simulink model "vehicle_longitudinal_model"  (Simulink 8.9)
settings: Solver=ode23s  StartTime=0.0  StopTime=10.0  RelTol=1e-3  EnableMultiTasking=on
values from neighbouring files (symbols this model uses):
  c_aero = 0.53    [Setup_Lincoln_model.m]
  delay_brake = 0.2    [Setup_Lincoln_model.m]
  F_roll = 172    [Setup_Lincoln_model.m]
  h = h_v    (= 0.33)    [Setup_Lincoln_model.m]
  I_e = 0.2630    (= 0.263)    [Setup_Lincoln_model.m]
  I_wheel = 1.93    [Setup_Lincoln_model.m]
  KB = 0.9    [Setup_Lincoln_model.m]
  mass = 2000    [Setup_Lincoln_model.m]
  max_throttle = max(throttle_table)    [Setup_Lincoln_model.m]
  max_throttle_rate = 450    [Setup_Lincoln_model.m]
  min_throttle = min(throttle_table)    [Setup_Lincoln_model.m]
  mu_B = 22+(Fz-1940)/645    (= 26.5968992248)    [Setup_Lincoln_model.m]
  mu_C = 1.35-(Fz-1940)/16125    (= 1.16612403101)    [Setup_Lincoln_model.m]
  mu_D = 2000+(Fz-1940)/0.956    (= 5101.46443515)    [Setup_Lincoln_model.m]
  mu_E = -3.6    [Setup_Lincoln_model.m]
  P_po = 10.67    [Setup_Lincoln_model.m]
  Rdrive = 0.3058    [Setup_Lincoln_model.m]
  tau_brake = 0.1    [Setup_Lincoln_model.m]
  tau_throttle = 0.01    [Setup_Lincoln_model.m]
  throttle_o = 2    [Setup_Lincoln_model.m]
  w_wheel_o = x_dot_o/he    (= 63.6363636364)    [Setup_Lincoln_model.m]
  we_max = max(we_table)    [Setup_Lincoln_model.m]
  we_min = min(we_table)    [Setup_Lincoln_model.m]
  we_o = x_dot_o/(he*Rdrive*gear_ratios(3))    [Setup_Lincoln_model.m]
  x_dot_o = 21    [Setup_Lincoln_model.m]
undefined symbols (not defined in the file or in its folder): tnet_table
libraries: simulink x2
settings Model: Creator=user  LastModifiedBy=edward
settings OptimizationCC: ExpressionDepthLimit=2147483647  InitFltsAndDblsToZero=on
settings DebuggingCC: SolverPrmCheckMsg=warning  FcnCallInpInsideContextMsg=error
settings GRTTargetCC: GeneratePreprocessorConditionals=Use local settings

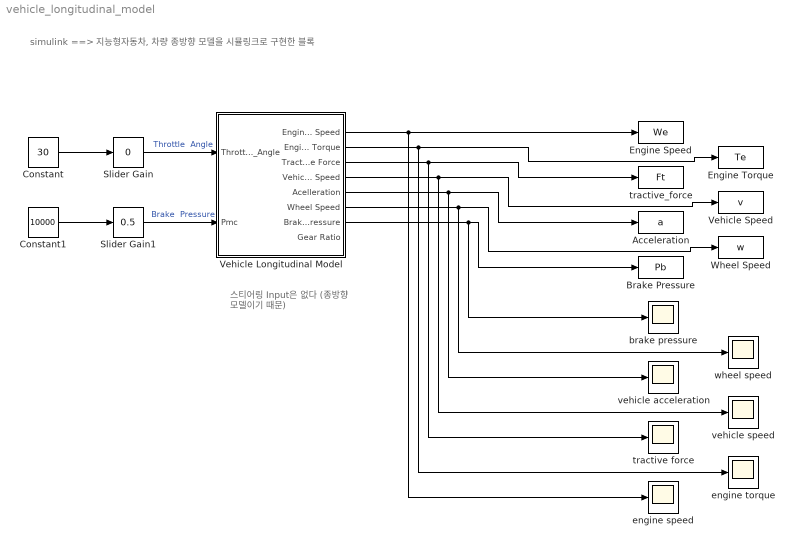
== system vehicle_longitudinal_model ==
  note: simulink ==> 지능형자동차, 차량 종방향 모델을 시뮬링크로 구현한 블록
  note: 스티어링 Input은 없다
      | (종방향 모델이기 때문)
  Acceleration : ToWorkspace  VariableName=a  SampleTime=-1
  Brake Pressure : ToWorkspace  VariableName=Pb  SampleTime=-1
  Constant : Constant  Value=30
  Constant1 : Constant  Value=10000
  Engine Speed : ToWorkspace  VariableName=We  SampleTime=-1
  Engine Torque : ToWorkspace  VariableName=Te  SampleTime=-1
  Slider Gain : simulink/Math Operations/Slider Gain  gain=0  low=0  high=1
  Slider Gain1 : simulink/Math Operations/Slider Gain  gain=0.5  low=0  high=1
  Vehicle Longitudinal Model : Subsystem
  Vehicle Speed : ToWorkspace  VariableName=v  SampleTime=-1
  Wheel Speed : ToWorkspace  VariableName=w  SampleTime=-1
  brake pressure : Scope
  engine speed : Scope
  engine torque : Scope
  tractive force : Scope
  tractive_force : ToWorkspace  VariableName=Ft  SampleTime=-1
  vehicle acceleration : Scope
  vehicle speed : Scope
  wheel speed : Scope
  wires:
  Constant/1 -> Slider Gain/1
  Slider Gain/1 -> Vehicle Longitudinal Model/1(Throttle_Angle)  "Throttle  Angle"
  Constant1/1 -> Slider Gain1/1
  Slider Gain1/1 -> Vehicle Longitudinal Model/2(Pmc)  "Brake  Pressure"
  Vehicle Longitudinal Model/1(Engine Speed) -> Engine Speed/1, engine speed/1
  Vehicle Longitudinal Model/3(Tractive Force) -> tractive force/1, tractive_force/1
  Vehicle Longitudinal Model/4(Vehicle Speed) -> Vehicle Speed/1, vehicle speed/1
  Vehicle Longitudinal Model/5(Acelleration) -> vehicle acceleration/1, Acceleration/1
  Vehicle Longitudinal Model/6(Wheel Speed) -> Wheel Speed/1, wheel speed/1
  Vehicle Longitudinal Model/7(Brake Pressure) -> brake pressure/1, Brake Pressure/1
  Vehicle Longitudinal Model/2(Engine Torque) -> Engine Torque/1, engine torque/1

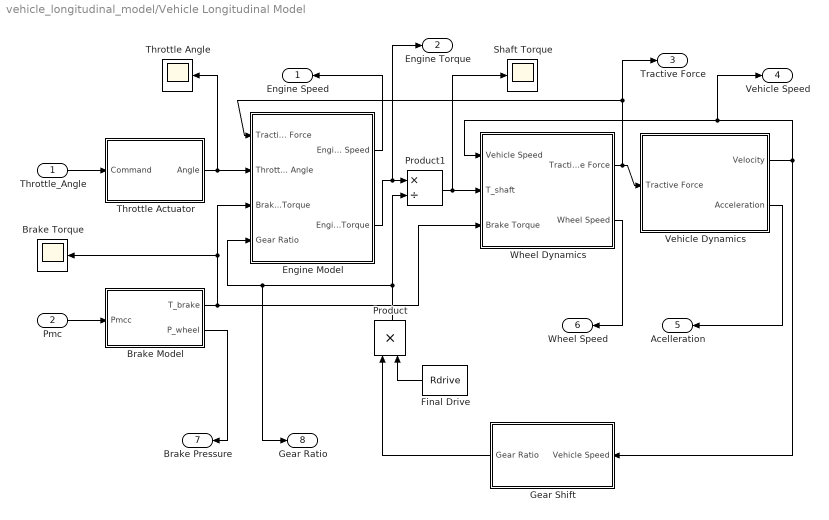
== system vehicle_longitudinal_model/Vehicle Longitudinal Model ==
  Throttle_Angle : Inport
  Pmc : Inport  Port=2
  Brake Model : Subsystem
  Brake Torque : Scope
  Engine Model : Subsystem
  Final Drive : Constant  Value=Rdrive
  Gear Shift : Subsystem
  Product : Product  Inputs=**  SaturateOnIntegerOverflow=on  RndMeth=Zero  InputSameDT=on  OutDataTypeStr=Inherit: Same as first input
  Product1 : Product  Inputs=*/  SaturateOnIntegerOverflow=on  RndMeth=Zero  InputSameDT=on  OutDataTypeStr=Inherit: Same as first input
  Shaft Torque : Scope
  Throttle Actuator : Subsystem
  Throttle Angle : Scope
  Vehicle Dynamics : Subsystem
  Wheel Dynamics : Subsystem
  Engine Speed : Outport
  Engine Torque : Outport  Port=2
  Tractive Force : Outport  Port=3
  Vehicle Speed : Outport  Port=4
  Acelleration : Outport  Port=5
  Wheel Speed : Outport  Port=6
  Brake Pressure : Outport  Port=7
  Gear Ratio : Outport  Port=8
  wires:
  Product1/1 -> Shaft Torque/1, Wheel Dynamics/2(T_shaft)
  Engine Model/2(Engine Torque) -> Product1/1, Engine Torque/1
  Engine Model/1(Engine Speed) -> Engine Speed/1
  Brake Model/1(T_brake) -> Engine Model/3(Brake Torque), Brake Torque/1, Wheel Dynamics/3(Brake Torque)
  Product/1 -> Product1/2, Engine Model/4(Gear Ratio), Gear Ratio/1
  Final Drive/1 -> Product/2
  Gear Shift/1(Gear Ratio) -> Product/1
  Wheel Dynamics/1(Tractive Force) -> Vehicle Dynamics/1(Tractive Force), Engine Model/1(Tractive Force), Tractive Force/1
  Throttle Actuator/1(Angle) -> Engine Model/2(Throttle Angle), Throttle Angle/1
  Throttle_Angle/1 -> Throttle Actuator/1(Command)
  Pmc/1 -> Brake Model/1(Pmcc)
  Brake Model/2(P_wheel) -> Brake Pressure/1
  Vehicle Dynamics/1(Velocity) -> Vehicle Speed/1, Wheel Dynamics/1(Vehicle Speed), Gear Shift/1(Vehicle Speed)
  Vehicle Dynamics/2(Acceleration) -> Acelleration/1
  Wheel Dynamics/2(Wheel Speed) -> Wheel Speed/1

== system vehicle_longitudinal_model/Vehicle Longitudinal Model/Brake Model ==
  note: Wheel Pressure가 브레이크 패드에 있는
      | Spring(k)보다 크게 걸렸을 때에만 브레이크가 작동하므로
      | Dead Zone이 발생한다
  note: Wheel pressure
  note: brake는 1차 전달함수의 response를 보인다
  note: Valve를 여닫는 시간에 따라
      | 필연적으로 발생하는 Time Delay
  Pmcc : Inport
  Brake Coefficient : Gain  Gain=KB  SaturateOnIntegerOverflow=on  OutDataTypeStr=Inherit: Same as input  ParamDataTypeStr=Inherit: Same as input
  Brake Dynamics : TransferFcn  Denominator=[tau_brake 1]
  Dead Zone : DeadZone  LowerValue=-P_po  UpperValue=P_po  SaturateOnIntegerOverflow=on
  Pure Time Delay : TransportDelay  DelayTime=delay_brake
  T_brake : Outport
  P_wheel : Outport  Port=2
  wires:
  Brake Coefficient/1 -> T_brake/1
  Dead Zone/1 -> Brake Coefficient/1
  Brake Dynamics/1 -> P_wheel/1, Dead Zone/1  "P_wheel"
  Pmcc/1 -> Pure Time Delay/1
  Pure Time Delay/1 -> Brake Dynamics/1

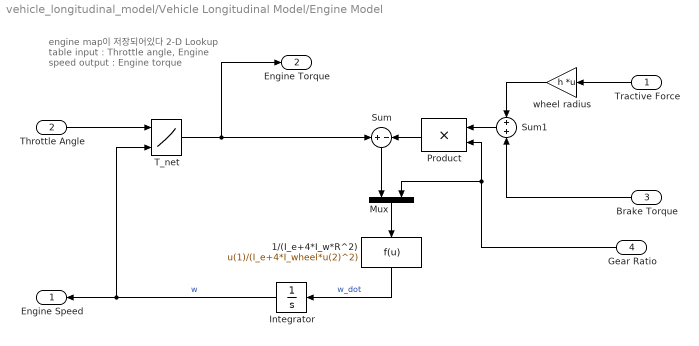
== system vehicle_longitudinal_model/Vehicle Longitudinal Model/Engine Model ==
  note: engine map이 저장되어있다
      | 2-D Lookup table
      |
      | input : Throttle angle, Engine speed
      | output : Engine torque
  Tractive Force : Inport
  Throttle Angle : Inport  Port=2
  Brake Torque : Inport  Port=3
  Gear Ratio : Inport  Port=4
  1/(I_e+4*I_w*R^2) : Fcn  Expr=u(1)/(I_e+4*I_wheel*u(2)^2)
  Integrator : Integrator  InitialCondition=we_o  LimitOutput=on  UpperSaturationLimit=[we_max]  LowerSaturationLimit=[we_min]
  Mux : Mux  Inputs=2
  Product : Product  SaturateOnIntegerOverflow=on  RndMeth=Zero  InputSameDT=on  OutDataTypeStr=Inherit: Same as first input
  Sum : Sum  Inputs=+|-  SaturateOnIntegerOverflow=on  InputSameDT=on  OutDataTypeStr=Inherit: Same as first input
  Sum1 : Sum  SaturateOnIntegerOverflow=on  InputSameDT=on  OutDataTypeStr=Inherit: Same as first input
  T_net : Lookup2D  RowIndex=alpha_table  ColumnIndex=we_table  Table=tnet_table  SaturateOnIntegerOverflow=on  InputSameDT=on
  wheel radius : Gain  Gain=h  Multiplication=Matrix(K*u)  SaturateOnIntegerOverflow=on  OutDataTypeStr=Inherit: Same as input  ParamDataTypeStr=Inherit: Same as input
  Engine Speed : Outport
  Engine Torque : Outport  Port=2
  wires:
  Throttle Angle/1 -> T_net/1
  Integrator/1 -> Engine Speed/1, T_net/2  "w"
  1/(I_e+4*I_w*R^2)/1 -> Integrator/1  "w_dot"
  Tractive Force/1 -> wheel radius/1
  wheel radius/1 -> Sum1/1
  Brake Torque/1 -> Sum1/2
  Product/1 -> Sum/2
  Sum1/1 -> Product/1
  Gear Ratio/1 -> Product/2, Mux/2
  Sum/1 -> Mux/1
  Mux/1 -> 1/(I_e+4*I_w*R^2)/1
  T_net/1 -> Engine Torque/1, Sum/1

== system vehicle_longitudinal_model/Vehicle Longitudinal Model/Gear Shift ==
  note: [1 1 1]인 [n,1] 행렬과
      | 반환행렬을 곱해서
      | 스칼라값(기어값)을 만든다
  note: 현재 차량 속도 vs 기어변속 속도를 비교한다
      | [0; 1; 1] 같은 [1,n]행렬이 반환된다
  Vehicle Speed : Inport
  Convert m/s to mph : Gain  Gain=3.6/1.6  SaturateOnIntegerOverflow=on  OutDataTypeStr=Inherit: Same as input  ParamDataTypeStr=Inherit: Same as input
  Direct Look-Up of Gear ratio : LookupNDDirect  NumberOfTableDimensions=1  Table=[0.3423,0.6378,1.0,1.4184]
  Get gear-1 : Gain  Gain=ones(1,3)  Multiplication=Matrix(K*u)  SaturateOnIntegerOverflow=on  OutDataTypeStr=Inherit: Same as input  ParamDataTypeStr=Inherit: Same as input
  Relational Operator : RelationalOperator  Operator=>  RndMeth=Nearest  InputSameDT=on
  Shift Speeds : Constant  Value=[15 32 67]
  Gear Ratio : Outport
  wires:
  Shift Speeds/1 -> Relational Operator/2
  Relational Operator/1 -> Get gear-1/1
  Convert m/s to mph/1 -> Relational Operator/1
  Get gear-1/1 -> Direct Look-Up of Gear ratio/1
  Vehicle Speed/1 -> Convert m/s to mph/1
  Direct Look-Up of Gear ratio/1 -> Gear Ratio/1

== system vehicle_longitudinal_model/Vehicle Longitudinal Model/Throttle Actuator ==
  Command : Inport
  Integrator : Integrator  InitialCondition=throttle_o  LimitOutput=on  UpperSaturationLimit=max_throttle  LowerSaturationLimit=min_throttle
  Saturation : Saturate  UpperLimit=max_throttle_rate  LowerLimit=-max_throttle_rate
  Sum : Sum  Inputs=-+|  SaturateOnIntegerOverflow=on  InputSameDT=on  OutDataTypeStr=Inherit: Same as first input
  Throttle Time Constant : Gain  Gain=1/tau_throttle  SaturateOnIntegerOverflow=on  OutDataTypeStr=Inherit: Same as input  ParamDataTypeStr=Inherit: Same as input
  Angle : Outport
  wires:
  Command/1 -> Sum/2
  Integrator/1 -> Angle/1, Sum/1
  Sum/1 -> Throttle Time Constant/1
  Throttle Time Constant/1 -> Saturation/1
  Saturation/1 -> Integrator/1

== system vehicle_longitudinal_model/Vehicle Longitudinal Model/Vehicle Dynamics ==
  note: 타이어저항 F_road
  note: v
  note: v_dot
  note: 공기저항 F_air
  note: 구름저항 F_roll
  Tractive Force : Inport
  Aerodynamic Drag : Fcn  Expr=c_aero*u^2
  Divide by Mass : Gain  Gain=1/mass  Multiplication=Matrix(K*u)  SaturateOnIntegerOverflow=on  OutDataTypeStr=Inherit: Same as input  ParamDataTypeStr=Inherit: Same as input
  Integrator : Integrator  InitialCondition=x_dot_o  LimitOutput=on  LowerSaturationLimit=0
  Rolling Resistance : Constant  Value=F_roll
  Sum1 : Sum  Inputs=--+  SaturateOnIntegerOverflow=on  InputSameDT=on  OutDataTypeStr=Inherit: Same as first input
  Velocity : Outport
  Acceleration : Outport  Port=2
  wires:
  Tractive Force/1 -> Sum1/3
  Divide by Mass/1 -> Acceleration/1, Integrator/1
  Integrator/1 -> Velocity/1, Aerodynamic Drag/1
  Sum1/1 -> Divide by Mass/1
  Rolling Resistance/1 -> Sum1/2
  Aerodynamic Drag/1 -> Sum1/1

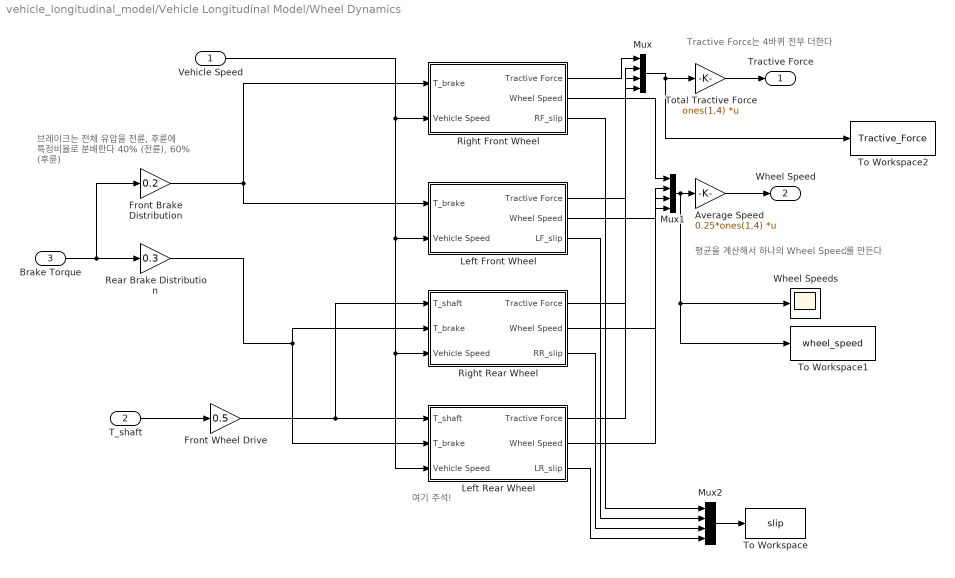
== system vehicle_longitudinal_model/Vehicle Longitudinal Model/Wheel Dynamics ==
  note: 여기 주석!
  note: Tractive Force는 4바퀴 전부 더한다
  note: 평균을 계산해서 하나의 Wheel Speed를 만든다
  note: 브레이크는 전체 유압을
      | 전륜, 후륜에 특정비율로 분배한다
      | 40% (전륜), 60% (후륜)
  Vehicle Speed : Inport
  T_shaft : Inport  Port=2
  Brake Torque : Inport  Port=3
  Average Speed : Gain  Gain=0.25*ones(1,4)  Multiplication=Matrix(K*u)  SaturateOnIntegerOverflow=on  OutDataTypeStr=Inherit: Same as input  ParamDataTypeStr=Inherit: Same as input
  Front Brake Distribution : Gain  Gain=0.2  SaturateOnIntegerOverflow=on  OutDataTypeStr=Inherit: Same as input  ParamDataTypeStr=Inherit: Same as input
  Front Wheel Drive : Gain  Gain=0.5  SaturateOnIntegerOverflow=on  OutDataTypeStr=Inherit: Same as input  ParamDataTypeStr=Inherit: Same as input
  Left Front Wheel : Subsystem
  Left Rear Wheel : Subsystem
  Mux : Mux
  Mux1 : Mux
  Mux2 : Mux
  Rear Brake Distribution : Gain  Gain=0.3  SaturateOnIntegerOverflow=on  OutDataTypeStr=Inherit: Same as input  ParamDataTypeStr=Inherit: Same as input
  Right Front Wheel : Subsystem
  Right Rear Wheel : Subsystem
  To Workspace : ToWorkspace  VariableName=slip  SampleTime=-1
  To Workspace1 : ToWorkspace  VariableName=wheel_speed  SampleTime=-1
  To Workspace2 : ToWorkspace  VariableName=Tractive_Force  SampleTime=-1
  Total Tractive Force : Gain  Gain=ones(1,4)  Multiplication=Matrix(K*u)  SaturateOnIntegerOverflow=on  OutDataTypeStr=Inherit: Same as input  ParamDataTypeStr=Inherit: Same as input
  Wheel Speeds : Scope
  Tractive Force : Outport
  Wheel Speed : Outport  Port=2
  wires:
  Total Tractive Force/1 -> Tractive Force/1
  Average Speed/1 -> Wheel Speed/1
  Mux/1 -> Total Tractive Force/1, To Workspace2/1
  Vehicle Speed/1 -> Right Front Wheel/2(Vehicle Speed), Left Rear Wheel/3(Vehicle Speed), Right Rear Wheel/3(Vehicle Speed), Left Front Wheel/2(Vehicle Speed)
  Right Front Wheel/1(Tractive Force) -> Mux/1
  Left Front Wheel/1(Tractive Force) -> Mux/2
  Right Rear Wheel/1(Tractive Force) -> Mux/3
  Left Rear Wheel/1(Tractive Force) -> Mux/4
  Mux1/1 -> Average Speed/1, Wheel Speeds/1, To Workspace1/1
  Right Front Wheel/2(Wheel Speed) -> Mux1/1
  Left Front Wheel/2(Wheel Speed) -> Mux1/2
  Right Rear Wheel/2(Wheel Speed) -> Mux1/3
  Left Rear Wheel/2(Wheel Speed) -> Mux1/4
  Right Front Wheel/3(RF_slip) -> Mux2/1
  Left Rear Wheel/3(LR_slip) -> Mux2/4
  Mux2/1 -> To Workspace/1
  T_shaft/1 -> Front Wheel Drive/1
  Front Wheel Drive/1 -> Right Rear Wheel/1(T_shaft), Left Rear Wheel/1(T_shaft)
  Brake Torque/1 -> Rear Brake Distribution/1, Front Brake Distribution/1
  Left Front Wheel/3(LF_slip) -> Mux2/2
  Right Rear Wheel/3(RR_slip) -> Mux2/3
  Front Brake Distribution/1 -> Right Front Wheel/1(T_brake), Left Front Wheel/1(T_brake)
  Rear Brake Distribution/1 -> Left Rear Wheel/2(T_brake), Right Rear Wheel/2(T_brake)

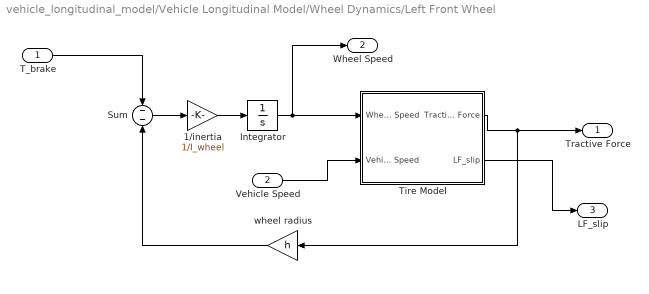
== system vehicle_longitudinal_model/Vehicle Longitudinal Model/Wheel Dynamics/Left Front Wheel ==
  T_brake : Inport
  Vehicle Speed : Inport  Port=2
  1/inertia : Gain  Gain=1/I_wheel  SaturateOnIntegerOverflow=on  OutDataTypeStr=Inherit: Same as input  ParamDataTypeStr=Inherit: Same as input
  Integrator : Integrator  InitialCondition=w_wheel_o
  Sum : Sum  Inputs=-|-  SaturateOnIntegerOverflow=on  InputSameDT=on  OutDataTypeStr=Inherit: Same as first input
  Tire Model : Subsystem
  wheel radius : Gain  Gain=h  SaturateOnIntegerOverflow=on  OutDataTypeStr=Inherit: Same as input  ParamDataTypeStr=Inherit: Same as input
  Tractive Force : Outport
  Wheel Speed : Outport  Port=2
  LF_slip : Outport  Port=3
  wires:
  1/inertia/1 -> Integrator/1
  Sum/1 -> 1/inertia/1
  Integrator/1 -> Wheel Speed/1, Tire Model/1(Wheel Speed)
  T_brake/1 -> Sum/1
  wheel radius/1 -> Sum/2
  Vehicle Speed/1 -> Tire Model/2(Vehicle Speed)
  Tire Model/1(Tractive Force) -> Tractive Force/1, wheel radius/1
  Tire Model/2(LF_slip) -> LF_slip/1

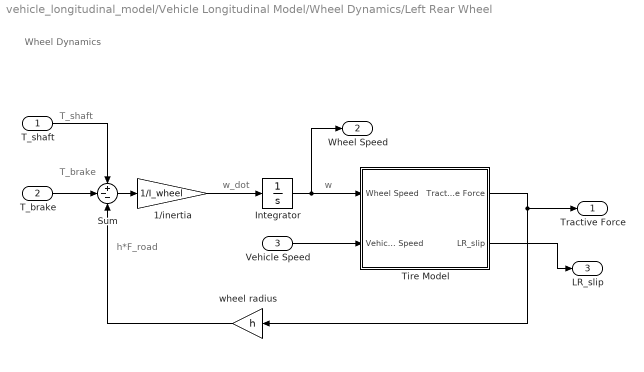
== system vehicle_longitudinal_model/Vehicle Longitudinal Model/Wheel Dynamics/Left Rear Wheel ==
  note: Wheel Dynamics
  note: h*F_road
  note: T_brake
  note: T_shaft
  note: w
  note: w_dot
  T_shaft : Inport
  T_brake : Inport  Port=2
  Vehicle Speed : Inport  Port=3
  1/inertia : Gain  Gain=1/I_wheel  SaturateOnIntegerOverflow=on  OutDataTypeStr=Inherit: Same as input  ParamDataTypeStr=Inherit: Same as input
  Integrator : Integrator  InitialCondition=w_wheel_o
  Sum : Sum  Inputs=+--  SaturateOnIntegerOverflow=on  InputSameDT=on  OutDataTypeStr=Inherit: Same as first input
  Tire Model : Subsystem
  wheel radius : Gain  Gain=h  SaturateOnIntegerOverflow=on  OutDataTypeStr=Inherit: Same as input  ParamDataTypeStr=Inherit: Same as input
  Tractive Force : Outport
  Wheel Speed : Outport  Port=2
  LR_slip : Outport  Port=3
  wires:
  1/inertia/1 -> Integrator/1
  Sum/1 -> 1/inertia/1
  Integrator/1 -> Wheel Speed/1, Tire Model/1(Wheel Speed)
  Vehicle Speed/1 -> Tire Model/2(Vehicle Speed)
  Tire Model/1(Tractive Force) -> Tractive Force/1, wheel radius/1
  Tire Model/2(LR_slip) -> LR_slip/1
  T_shaft/1 -> Sum/1
  T_brake/1 -> Sum/2
  wheel radius/1 -> Sum/3

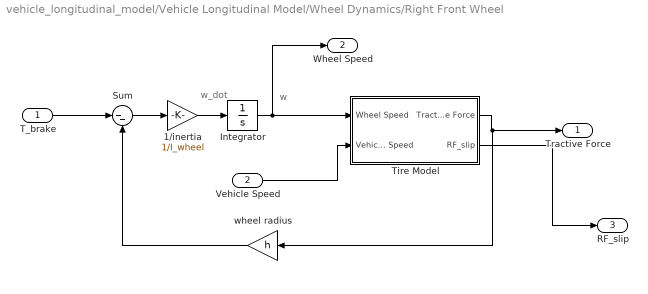
== system vehicle_longitudinal_model/Vehicle Longitudinal Model/Wheel Dynamics/Right Front Wheel ==
  note: w
  note: w_dot
  T_brake : Inport
  Vehicle Speed : Inport  Port=2
  1/inertia : Gain  Gain=1/I_wheel  SaturateOnIntegerOverflow=on  OutDataTypeStr=Inherit: Same as input  ParamDataTypeStr=Inherit: Same as input
  Integrator : Integrator  InitialCondition=w_wheel_o
  Sum : Sum  Inputs=|--  SaturateOnIntegerOverflow=on  InputSameDT=on  OutDataTypeStr=Inherit: Same as first input
  Tire Model : Subsystem
  wheel radius : Gain  Gain=h  SaturateOnIntegerOverflow=on  OutDataTypeStr=Inherit: Same as input  ParamDataTypeStr=Inherit: Same as input
  Tractive Force : Outport
  Wheel Speed : Outport  Port=2
  RF_slip : Outport  Port=3
  wires:
  1/inertia/1 -> Integrator/1
  Sum/1 -> 1/inertia/1
  Integrator/1 -> Wheel Speed/1, Tire Model/1(Wheel Speed)
  Vehicle Speed/1 -> Tire Model/2(Vehicle Speed)
  Tire Model/1(Tractive Force) -> Tractive Force/1, wheel radius/1
  Tire Model/2(RF_slip) -> RF_slip/1
  wheel radius/1 -> Sum/2
  T_brake/1 -> Sum/1

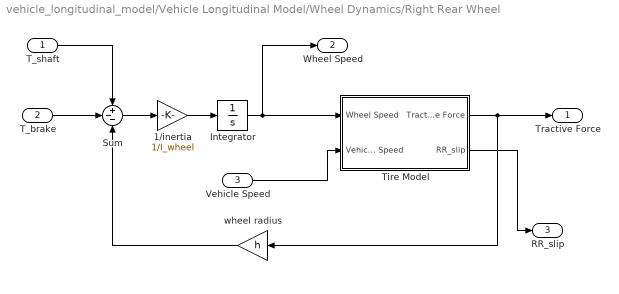
== system vehicle_longitudinal_model/Vehicle Longitudinal Model/Wheel Dynamics/Right Rear Wheel ==
  T_shaft : Inport
  T_brake : Inport  Port=2
  Vehicle Speed : Inport  Port=3
  1/inertia : Gain  Gain=1/I_wheel  SaturateOnIntegerOverflow=on  OutDataTypeStr=Inherit: Same as input  ParamDataTypeStr=Inherit: Same as input
  Integrator : Integrator  InitialCondition=w_wheel_o
  Sum : Sum  Inputs=+--  SaturateOnIntegerOverflow=on  InputSameDT=on  OutDataTypeStr=Inherit: Same as first input
  Tire Model : Subsystem
  wheel radius : Gain  Gain=h  SaturateOnIntegerOverflow=on  OutDataTypeStr=Inherit: Same as input  ParamDataTypeStr=Inherit: Same as input
  Tractive Force : Outport
  Wheel Speed : Outport  Port=2
  RR_slip : Outport  Port=3
  wires:
  1/inertia/1 -> Integrator/1
  Sum/1 -> 1/inertia/1
  Integrator/1 -> Wheel Speed/1, Tire Model/1(Wheel Speed)
  Vehicle Speed/1 -> Tire Model/2(Vehicle Speed)
  Tire Model/1(Tractive Force) -> Tractive Force/1, wheel radius/1
  Tire Model/2(RR_slip) -> RR_slip/1
  T_brake/1 -> Sum/2
  wheel radius/1 -> Sum/3
  T_shaft/1 -> Sum/1

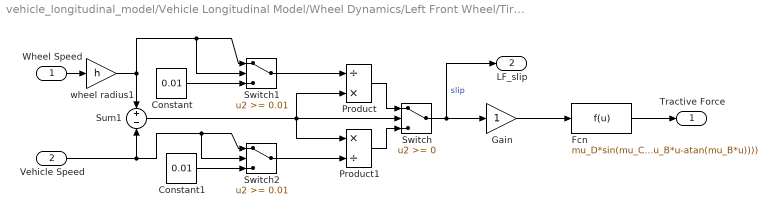
== system vehicle_longitudinal_model/Vehicle Longitudinal Model/Wheel Dynamics/Left Front Wheel/Tire Model ==
  Wheel Speed : Inport
  Vehicle Speed : Inport  Port=2
  Constant : Constant  Value=0.01
  Constant1 : Constant  Value=0.01
  Fcn : Fcn  Expr=mu_D*sin(mu_C*atan(mu_B*u-mu_E*(mu_B*u-atan(mu_B*u))))
  Gain : Gain  SaturateOnIntegerOverflow=on  OutDataTypeStr=Inherit: Same as input  ParamDataTypeStr=Inherit: Same as input
  Product : Product  Inputs=/*  SaturateOnIntegerOverflow=on  RndMeth=Zero  InputSameDT=on  OutDataTypeStr=Inherit: Same as first input
  Product1 : Product  Inputs=*/  SaturateOnIntegerOverflow=on  RndMeth=Zero  InputSameDT=on  OutDataTypeStr=Inherit: Same as first input
  Sum1 : Sum  Inputs=+-  SaturateOnIntegerOverflow=on  InputSameDT=on  OutDataTypeStr=Inherit: Same as first input
  Switch : Switch  SaturateOnIntegerOverflow=on  InputSameDT=on
  Switch1 : Switch  Threshold=0.01  SaturateOnIntegerOverflow=on  InputSameDT=on
  Switch2 : Switch  Threshold=0.01  SaturateOnIntegerOverflow=on  InputSameDT=on
  wheel radius1 : Gain  Gain=h  SaturateOnIntegerOverflow=on  OutDataTypeStr=Inherit: Same as input  ParamDataTypeStr=Inherit: Same as input
  Tractive Force : Outport
  LF_slip : Outport  Port=2
  wires:
  wheel radius1/1 -> Sum1/1, Switch1/1, Switch1/2
  Sum1/1 -> Switch/2, Product/2, Product1/1
  Product/1 -> Switch/1
  Product1/1 -> Switch/3
  Switch/1 -> Gain/1, LF_slip/1  "slip"
  Wheel Speed/1 -> wheel radius1/1
  Fcn/1 -> Tractive Force/1
  Vehicle Speed/1 -> Sum1/2, Switch2/1, Switch2/2
  Gain/1 -> Fcn/1
  Constant/1 -> Switch1/3
  Switch1/1 -> Product/1
  Switch2/1 -> Product1/2
  Constant1/1 -> Switch2/3

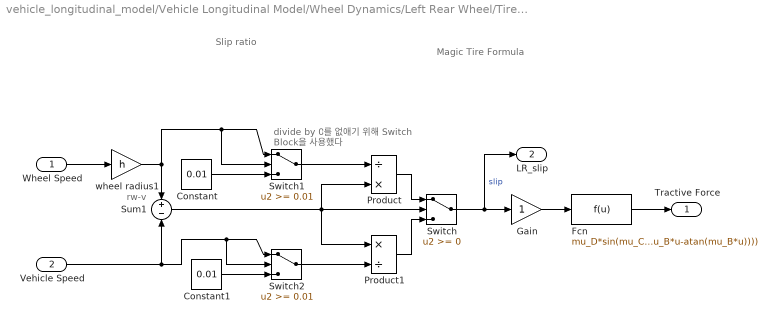
== system vehicle_longitudinal_model/Vehicle Longitudinal Model/Wheel Dynamics/Left Rear Wheel/Tire Model ==
  note: Magic Tire Formula
  note: rw-v
  note: Slip ratio
  note: divide by 0를 없애기 위해
      | Switch Block을 사용했다
  Wheel Speed : Inport
  Vehicle Speed : Inport  Port=2
  Constant : Constant  Value=0.01
  Constant1 : Constant  Value=0.01
  Fcn : Fcn  Expr=mu_D*sin(mu_C*atan(mu_B*u-mu_E*(mu_B*u-atan(mu_B*u))))
  Gain : Gain  SaturateOnIntegerOverflow=on  OutDataTypeStr=Inherit: Same as input  ParamDataTypeStr=Inherit: Same as input
  Product : Product  Inputs=/*  SaturateOnIntegerOverflow=on  RndMeth=Zero  InputSameDT=on  OutDataTypeStr=Inherit: Same as first input
  Product1 : Product  Inputs=*/  SaturateOnIntegerOverflow=on  RndMeth=Zero  InputSameDT=on  OutDataTypeStr=Inherit: Same as first input
  Sum1 : Sum  Inputs=+-  SaturateOnIntegerOverflow=on  InputSameDT=on  OutDataTypeStr=Inherit: Same as first input
  Switch : Switch  SaturateOnIntegerOverflow=on  InputSameDT=on
  Switch1 : Switch  Threshold=0.01  SaturateOnIntegerOverflow=on  InputSameDT=on
  Switch2 : Switch  Threshold=0.01  SaturateOnIntegerOverflow=on  InputSameDT=on
  wheel radius1 : Gain  Gain=h  SaturateOnIntegerOverflow=on  OutDataTypeStr=Inherit: Same as input  ParamDataTypeStr=Inherit: Same as input
  Tractive Force : Outport
  LR_slip : Outport  Port=2
  wires:
  wheel radius1/1 -> Sum1/1, Switch1/1, Switch1/2
  Sum1/1 -> Switch/2, Product/2, Product1/1
  Product/1 -> Switch/1
  Product1/1 -> Switch/3
  Switch/1 -> Gain/1, LR_slip/1  "slip"
  Wheel Speed/1 -> wheel radius1/1
  Fcn/1 -> Tractive Force/1
  Vehicle Speed/1 -> Sum1/2, Switch2/1, Switch2/2
  Gain/1 -> Fcn/1
  Constant/1 -> Switch1/3
  Switch1/1 -> Product/1
  Switch2/1 -> Product1/2
  Constant1/1 -> Switch2/3

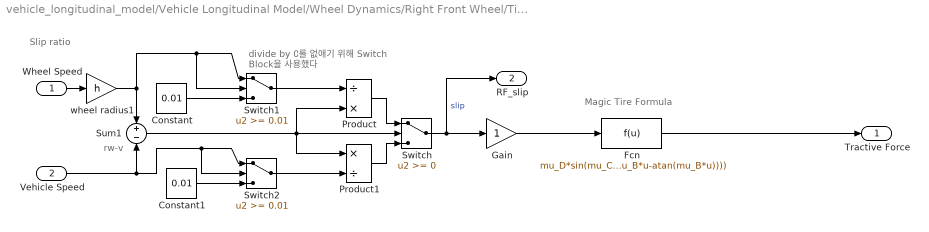
== system vehicle_longitudinal_model/Vehicle Longitudinal Model/Wheel Dynamics/Right Front Wheel/Tire Model ==
  note: rw-v
  note: Magic Tire Formula
  note: Slip ratio
  note: divide by 0를 없애기 위해
      | Switch Block을 사용했다
  Wheel Speed : Inport
  Vehicle Speed : Inport  Port=2
  Constant : Constant  Value=0.01
  Constant1 : Constant  Value=0.01
  Fcn : Fcn  Expr=mu_D*sin(mu_C*atan(mu_B*u-mu_E*(mu_B*u-atan(mu_B*u))))
  Gain : Gain  SaturateOnIntegerOverflow=on  OutDataTypeStr=Inherit: Same as input  ParamDataTypeStr=Inherit: Same as input
  Product : Product  Inputs=/*  SaturateOnIntegerOverflow=on  RndMeth=Zero  InputSameDT=on  OutDataTypeStr=Inherit: Same as first input
  Product1 : Product  Inputs=*/  SaturateOnIntegerOverflow=on  RndMeth=Zero  InputSameDT=on  OutDataTypeStr=Inherit: Same as first input
  Sum1 : Sum  Inputs=+-  SaturateOnIntegerOverflow=on  InputSameDT=on  OutDataTypeStr=Inherit: Same as first input
  Switch : Switch  SaturateOnIntegerOverflow=on  InputSameDT=on
  Switch1 : Switch  Threshold=0.01  SaturateOnIntegerOverflow=on  InputSameDT=on
  Switch2 : Switch  Threshold=0.01  SaturateOnIntegerOverflow=on  InputSameDT=on
  wheel radius1 : Gain  Gain=h  SaturateOnIntegerOverflow=on  OutDataTypeStr=Inherit: Same as input  ParamDataTypeStr=Inherit: Same as input
  Tractive Force : Outport
  RF_slip : Outport  Port=2
  wires:
  wheel radius1/1 -> Sum1/1, Switch1/1, Switch1/2
  Sum1/1 -> Switch/2, Product/2, Product1/1
  Product/1 -> Switch/1
  Product1/1 -> Switch/3
  Switch/1 -> Gain/1, RF_slip/1  "slip"
  Wheel Speed/1 -> wheel radius1/1
  Fcn/1 -> Tractive Force/1
  Vehicle Speed/1 -> Sum1/2, Switch2/1, Switch2/2
  Gain/1 -> Fcn/1
  Constant/1 -> Switch1/3
  Switch1/1 -> Product/1
  Switch2/1 -> Product1/2
  Constant1/1 -> Switch2/3

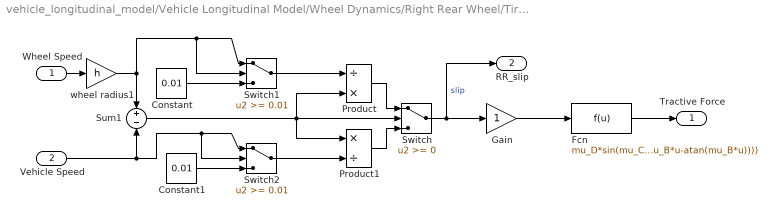
== system vehicle_longitudinal_model/Vehicle Longitudinal Model/Wheel Dynamics/Right Rear Wheel/Tire Model ==
  Wheel Speed : Inport
  Vehicle Speed : Inport  Port=2
  Constant : Constant  Value=0.01
  Constant1 : Constant  Value=0.01
  Fcn : Fcn  Expr=mu_D*sin(mu_C*atan(mu_B*u-mu_E*(mu_B*u-atan(mu_B*u))))
  Gain : Gain  SaturateOnIntegerOverflow=on  OutDataTypeStr=Inherit: Same as input  ParamDataTypeStr=Inherit: Same as input
  Product : Product  Inputs=/*  SaturateOnIntegerOverflow=on  RndMeth=Zero  InputSameDT=on  OutDataTypeStr=Inherit: Same as first input
  Product1 : Product  Inputs=*/  SaturateOnIntegerOverflow=on  RndMeth=Zero  InputSameDT=on  OutDataTypeStr=Inherit: Same as first input
  Sum1 : Sum  Inputs=+-  SaturateOnIntegerOverflow=on  InputSameDT=on  OutDataTypeStr=Inherit: Same as first input
  Switch : Switch  SaturateOnIntegerOverflow=on  InputSameDT=on
  Switch1 : Switch  Threshold=0.01  SaturateOnIntegerOverflow=on  InputSameDT=on
  Switch2 : Switch  Threshold=0.01  SaturateOnIntegerOverflow=on  InputSameDT=on
  wheel radius1 : Gain  Gain=h  SaturateOnIntegerOverflow=on  OutDataTypeStr=Inherit: Same as input  ParamDataTypeStr=Inherit: Same as input
  Tractive Force : Outport
  RR_slip : Outport  Port=2
  wires:
  wheel radius1/1 -> Sum1/1, Switch1/1, Switch1/2
  Sum1/1 -> Switch/2, Product/2, Product1/1
  Product/1 -> Switch/1
  Product1/1 -> Switch/3
  Switch/1 -> Gain/1, RR_slip/1  "slip"
  Wheel Speed/1 -> wheel radius1/1
  Fcn/1 -> Tractive Force/1
  Vehicle Speed/1 -> Sum1/2, Switch2/1, Switch2/2
  Gain/1 -> Fcn/1
  Constant/1 -> Switch1/3
  Switch1/1 -> Product/1
  Switch2/1 -> Product1/2
  Constant1/1 -> Switch2/3
